simulink model "probm5"  (R2020a)
settings: Solver=VariableStepAuto  StartTime=0.0  StopTime=10.0  RelTol=1e-3
model workspace (MAT data in the model file):
  C = Simulink.Parameter
  C.Value = 1e-05
  C.DataType = 'auto'
  C.Dimensions = [1 1]
  R = Simulink.Parameter
  R.Value = 10
  R.DataType = 'auto'
  R.Dimensions = [1 1]
settings Model: Creator=DELL  LastModifiedBy=DELL

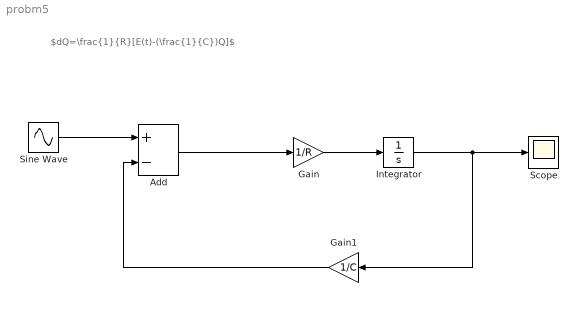
== system probm5 ==
  note: $dQ=\frac{1}{R}[E(t)-(\frac{1}{C})Q]$
  Add : Sum  Inputs=+-
  Gain : Gain  Gain=1/R
  Gain1 : Gain  Gain=1/C
  Integrator : Integrator
  Scope : Scope
  Sine Wave : Sin  Frequency=10  SampleTime=0
  wires:
  Gain1/1 -> Add/2
  Integrator/1 -> Gain1/1, Scope/1
  Gain/1 -> Integrator/1
  Sine Wave/1 -> Add/1
  Add/1 -> Gain/1
